simulink library "P45BPack_lib"  (R2025b)
settings: Solver=VariableStepAuto  StartTime=0.0  StopTime=10.0  RelTol=1e-3
values from neighbouring files (symbols this model uses):
  Np = evalin('base','Np')    [P45B.m]
  Ns = evalin('base','Ns')    [P45B.m]
undefined symbols (not defined in the file or in its folder): battery_builder_rtmsupport, gcbh, ModuleType1, ParallelAssemblyType1
libraries: nesl_utility x1, $bdroot x1
settings Model: Creator=nhamb  LastModifiedBy=nhamb

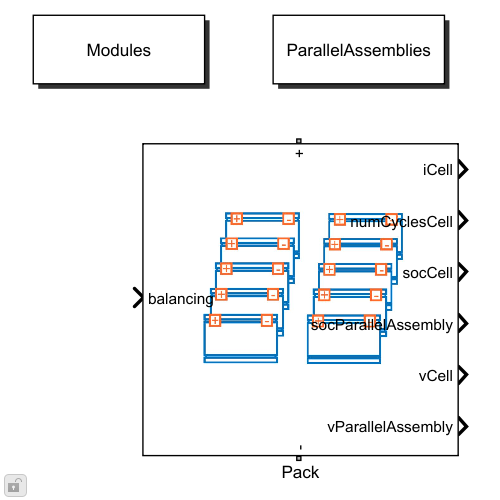
[thumbnail: Simulink's stored preview of the top-level diagram]
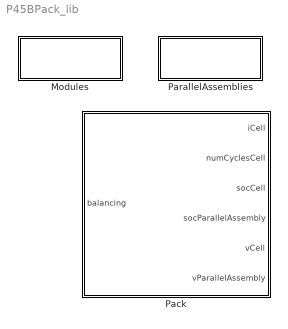
== system P45BPack_lib ==
  Modules : Subsystem  Tag=simscape_sublibrary
      mask Display: disp(get_param(gcb,'Name'))
  Pack : Subsystem  LoadFcn=battery_builder_rtmsupport('loadfcn',gcbh);
      settings: CopyFcn=battery_builder_rtmsupport('copyfcn',gcbh);  PreCopyFcn=battery_builder_rtmsupport('precopyfcn',gcbh);  PreDeleteFcn=battery_builder_rtmsupport('predeletefcn',gcbh);  PortSchema="{\"entries\":[{\"content\":{\"sides\":[{\"content\":{\"connectorIds\":[\"LConn1\"]},\"type\":\"ConnectorPlacement.EquallySpacedRectSide\",\"uuid\":\"bc69bedc-f021-4d63-9cf6-00df1ff9d80c\"},{\"content\":{\"connectorIds\":[\"RConn1\"],\"side\":\"RIGHT\"},\"type\":\"ConnectorPlacement.EquallySpacedRectSide\",\"uuid\":\"ae59a785-8ad2-4f04-8013-c306f8ca013b\"},{\"content\":{\"connectorIds\":[\"In1\"],\"side\":\"TOP\"},\"type\":\"ConnectorPlacement.EquallySpacedRectSide\",\"uuid\":\"2fb09327-c989-4719-8aff-5b8c99eb6fa6\"},{\"content\":{\"connectorIds\":[\"Out1\",\"Out2\",\"Out3\",\"Out4\",\"Out5\",\"Out6\"],\"side\":\"BOTTOM\"},\"type\":\"ConnectorPlacement.EquallySpacedRectSide\",\"uuid\":\"6b10cb86-7c8b-440d-835b-b9a65533e5ae\"}]},\"type\":\"ConnectorPlacement.EquallySpacedConnector\",\"uuid\":\"f3d89880-257d-496e-9c60-b9e40a370fad\"}],\"packageUris\":[\"http://schema.mathworks.com/mf0/Connector/R2020b\"],\"version\":\"1.0\"}"
      mask Display: image('$imagefile')
  ParallelAssemblies : Subsystem  Tag=simscape_sublibrary
      mask Display: disp(get_param(gcb,'Name'))

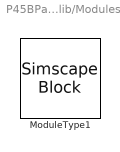
== system P45BPack_lib/Modules ==
  ModuleType1 : SimscapeBlock  DialogController=NetworkEngine.DynNeDlgSource  LoadFcn=|  SourceFile=P45BPack.Modules.ModuleType1  mask(ModuleType1){ComponentPath=P45BPack.Modules.ModuleType1, ComponentVariants=["P45BPack.Modules.ModuleType1"], ComponentVariantNames=["ModuleType1"], ClassName=ModuleType1, SchemaVersion=1, SOC_vecCell=ModuleType1.SOC_vecCell, SOC_vecCell_unit=1, SOC_vecCell_conf=compiletime, SOC_vecCellPercentDeviation=ModuleType1.SOC_vecCellPercentDeviation, SOC_vecCellPercentDeviation_unit=1, SOC_vecCellPercentDeviation_conf=compiletime, V0_vecCell=ModuleType1.V0_vecCell, V0_vecCell_unit=V, V0_vecCell_conf=compiletime, V0_vecCellPercentDeviation=ModuleType1.V0_vecCellPercentDeviation, V0_vecCellPercentDeviation_unit=1, V0_vecCellPercentDeviation_conf=compiletime, V_rangeCell=ModuleType1.V_rangeCell, V_rangeCell_unit=V, V_rangeCell_conf=compiletime, V_rangeCellPercentDeviation=ModuleType1.V_rangeCellPercentDeviation, V_rangeCellPercentDeviation_unit=1, V_rangeCellPercentDeviation_conf=compiletime, R0_vecCell=ModuleType1.R0_vecCell, R0_vecCell_unit=Ohm, R0_vecCell_conf=compiletime, R0_vecCellPercentDeviation=ModuleType1.R0_vecCellPercentDeviation, R0_vecCellPercentDeviation_unit=1, R0_vecCellPercentDeviation_conf=compiletime, AHCell=ModuleType1.AHCell, AHCell_unit=A*hr, AHCell_conf=compiletime, AHCellPercentDeviation=ModuleType1.AHCellPercentDeviation, AHCellPercentDeviation_unit=1, AHCellPercentDeviation_conf=compiletime, extrapolation_optionCell=simscape.enum.extrapolation.nearest, extrapolation_optionCell_unit=1, extrapolation_optionCell_conf=compiletime, R1_vecCell=ModuleType1.R1_vecCell, R1_vecCell_unit=Ohm, R1_vecCell_conf=compiletime, R1_vecCellPercentDeviation=ModuleType1.R1_vecCellPercentDeviation, R1_vecCellPercentDeviation_unit=1, R1_vecCellPercentDeviation_conf=compiletime, tau1_vecCell=ModuleType1.tau1_vecCell, tau1_vecCell_unit=s, tau1_vecCell_conf=compiletime, tau1_vecCellPercentDeviation=ModuleType1.tau1_vecCellPercentDeviation, tau1_vecCellPercentDeviation_unit=1, tau1_vecCellPercentDeviation_conf=compiletime, CellBalancingClosedResistance=ModuleType1.CellBalancingClosedResistance, CellBalancingClosedResistance_unit=Ohm, CellBalancingClosedResistance_conf=compiletime, CellBalancingOpenConductance=ModuleType1.CellBalancingOpenConductance, CellBalancingOpenConductance_unit=1/Ohm, CellBalancingOpenConductance_conf=compiletime, CellBalancingThreshold=ModuleType1.CellBalancingThreshold, CellBalancingThreshold_unit=1, CellBalancingThreshold_conf=compiletime, CellBalancingResistance=ModuleType1.CellBalancingResistance, CellBalancingResistance_unit=Ohm, CellBalancingResistance_conf=compiletime, P=2, P_unit=1, P_conf=compiletime, S=10, S_unit=1, S_conf=compiletime, iCell_specify=off, iCell_priority=None, iCell=repmat(0, 20, 1), iCell_unit=A, iCell_nominal_specify=off, iCell_nominal_value=1, iCell_nominal_unit=A, vCell_specify=off, vCell_priority=None, vCell=repmat(0, 20, 1), vCell_unit=V, vCell_nominal_specify=off, vCell_nominal_value=1, vCell_nominal_unit=V, socCell_specify=off, socCell_priority=High, socCell=repmat(1, 20, 1), socCell_unit=1, socCell_nominal_specify=off, socCell_nominal_value=1, socCell_nominal_unit=1, numCyclesCell_specify=off, numCyclesCell_priority=High, numCyclesCell=repmat(0, 20, 1), numCyclesCell_unit=1, numCyclesCell_nominal_specify=off, numCyclesCell_nominal_value=1, numCyclesCell_nominal_unit=1, vParallelAssembly_specify=off, vParallelAssembly_priority=None, vParallelAssembly=repmat(0, 10, 1), vParallelAssembly_unit=V, vParallelAssembly_nominal_specify=off, vParallelAssembly_nominal_value=1, vParallelAssembly_nominal_unit=V, socParallelAssembly_specify=off, socParallelAssembly_priority=None, socParallelAssembly=repmat(1, 10, 1), socParallelAssembly_unit=1, socParallelAssembly_nominal_specify=off, socParallelAssembly_nominal_value=1, socParallelAssembly_nominal_unit=1}
      | simscape.compiler.sli.internal.callback('LoadFcn',gcbh);
      | battery_builder_rtmsupport('loadfcn',gcbh);
      mask prompts: SOC_vecCell "Vector of state-of-charge values, SOC"; SOC_vecCellPercentDeviation "Percent deviation for SOC_vecCell"; V0_vecCell "Open-circuit voltage, V0(SOC)"; V0_vecCellPercentDeviation "Percent deviation for V0_vecCell"; V_rangeCell "Terminal voltage operating range [Min Max]"; V_rangeCellPercentDeviation "Percent deviation for V_rangeCell"; R0_vecCell "Terminal resistance, R0(SOC)"; R0_vecCellPercentDeviation "Percent deviation for R0_vecCell"; AHCell "Cell capacity, AH"; AHCellPercentDeviation "Percent deviation for AHCell"; extrapolation_optionCell "Extrapolation method for all tables"; R1_vecCell "First polarization resistance, R1(SOC)"; R1_vecCellPercentDeviation "Percent deviation for R1_vecCell"; tau1_vecCell "First time constant, tau1(SOC)"; tau1_vecCellPercentDeviation "Percent deviation for tau1_vecCell"; CellBalancingClosedResistance "Cell balancing switch closed resistance"; CellBalancingOpenConductance "Cell balancing switch open conductance"; CellBalancingThreshold "Cell balancing switch operation threshold"; CellBalancingResistance "Cell balancing shunt resistance"; P "Batteries in Parallel"; S "Batteries in Series"
      mask help:
      | Module Block
      |    Model resolution: Detailed
      |    Number of parallel assemblies: 10
      |    Number of cells per parallel assembly: 2
      |
      |    MATLAB version: 25.2
      |    Simscape Battery version: 25.2
      |    Simscape code generated on: 07-Sep-2026 17:43:40
      mask init:
      | simscape.compiler.sli.internal.preinitmask(gcb);
      settings: DeleteFcn=simscape.compiler.sli.internal.callback('DeleteFcn',gcbh);  ModelCloseFcn=simscape.compiler.sli.internal.callback('ModelCloseFcn',gcbh);  PreSaveFcn=simscape.compiler.sli.internal.callback('PreSaveFcn',gcbh);  PostSaveFcn=simscape.compiler.sli.internal.callback('PostSaveFcn',gcbh);  InternalSimscapePortConfiguration="{\"Bottom\":[{\"id\":\"n\",\"label\":\"-\",\"type\":\"foundation.electrical.electrical\"}],\"Left\":[{\"id\":\"enableCellBalancing\",\"label\":\"CB\",\"type\":\"input\"}],\"Right\":[],\"Top\":[{\"id\":\"p\",\"label\":\"+\",\"type\":\"foundation.electrical.electrical\"}]}"
      settings: CopyFcn=|
      | simscape.compiler.sli.internal.callback('CopyFcn',gcbh);
      | battery_builder_rtmsupport('copyfcn',gcbh);
      settings: PreCopyFcn=|
      | simscape.compiler.sli.internal.callback('PreCopyFcn',gcbh);
      | battery_builder_rtmsupport('precopyfcn',gcbh);
      settings: PreDeleteFcn=|
      | simscape.compiler.sli.internal.callback('PreDeleteFcn',gcbh);
      | battery_builder_rtmsupport('predeletefcn',gcbh);
      mask Help: web(nesl_help(gcbh))
      mask TypeOptions SOC_vecCell_unit: 1
      mask TypeOptions SOC_vecCell_conf: compiletime | runtime
      mask TypeOptions SOC_vecCellPercentDeviation_unit: 1
      mask TypeOptions SOC_vecCellPercentDeviation_conf: compiletime | runtime
      mask TypeOptions V0_vecCell_unit: V | MV | kV | mV
      mask TypeOptions V0_vecCell_conf: compiletime | runtime
      mask TypeOptions V0_vecCellPercentDeviation_unit: 1
      mask TypeOptions V0_vecCellPercentDeviation_conf: compiletime | runtime
      mask TypeOptions V_rangeCell_unit: V | MV | kV | mV
      mask TypeOptions V_rangeCell_conf: compiletime | runtime
      mask TypeOptions V_rangeCellPercentDeviation_unit: 1
      mask TypeOptions V_rangeCellPercentDeviation_conf: compiletime | runtime
      mask TypeOptions R0_vecCell_unit: Ohm | GOhm | MOhm | kOhm | mOhm
      mask TypeOptions R0_vecCell_conf: compiletime | runtime
      mask TypeOptions R0_vecCellPercentDeviation_unit: 1
      mask TypeOptions R0_vecCellPercentDeviation_conf: compiletime | runtime
      mask TypeOptions AHCell_unit: C | Ah | mC | nC | uC | MAh | kAh | mAh | A*hr
      mask TypeOptions AHCell_conf: compiletime | runtime
      mask TypeOptions AHCellPercentDeviation_unit: 1
      mask TypeOptions AHCellPercentDeviation_conf: compiletime | runtime
      mask TypeOptions extrapolation_optionCell: simscape.enum.extrapolation.linear | simscape.enum.extrapolation.nearest | simscape.enum.extrapolation.error
      mask TypeOptions extrapolation_optionCell_unit: 1
      mask TypeOptions extrapolation_optionCell_conf: compiletime
      mask TypeOptions R1_vecCell_unit: Ohm | GOhm | MOhm | kOhm | mOhm
      mask TypeOptions R1_vecCell_conf: compiletime | runtime
      mask TypeOptions R1_vecCellPercentDeviation_unit: 1
      mask TypeOptions R1_vecCellPercentDeviation_conf: compiletime | runtime
      mask TypeOptions tau1_vecCell_unit: d | s | hr | ms | ns | us | min
      mask TypeOptions tau1_vecCell_conf: compiletime | runtime
      mask TypeOptions tau1_vecCellPercentDeviation_unit: 1
      mask TypeOptions tau1_vecCellPercentDeviation_conf: compiletime | runtime
      mask TypeOptions CellBalancingClosedResistance_unit: Ohm | GOhm | MOhm | kOhm | mOhm
      mask TypeOptions CellBalancingClosedResistance_conf: compiletime | runtime
      mask TypeOptions CellBalancingOpenConductance_unit: S | mS | nS | uS | 1/Ohm
      mask TypeOptions CellBalancingOpenConductance_conf: compiletime | runtime
      mask TypeOptions CellBalancingThreshold_unit: 1
      mask TypeOptions CellBalancingThreshold_conf: compiletime | runtime
      mask TypeOptions CellBalancingResistance_unit: Ohm | GOhm | MOhm | kOhm | mOhm
      mask TypeOptions CellBalancingResistance_conf: compiletime | runtime
      mask TypeOptions P_unit: 1
      mask TypeOptions P_conf: compiletime
      mask TypeOptions S_unit: 1
      mask TypeOptions S_conf: compiletime
      mask TypeOptions iCell_priority: None | Low | High
      mask TypeOptions iCell_unit: A | MA | kA | mA | nA | pA | uA
      mask TypeOptions iCell_nominal_unit: A | MA | kA | mA | nA | pA | uA
      mask TypeOptions vCell_priority: None | Low | High
      mask TypeOptions vCell_unit: V | MV | kV | mV
      mask TypeOptions vCell_nominal_unit: V | MV | kV | mV
      mask TypeOptions socCell_priority: None | Low | High
      mask TypeOptions socCell_unit: 1
      mask TypeOptions socCell_nominal_unit: 1
      mask TypeOptions numCyclesCell_priority: None | Low | High
      mask TypeOptions numCyclesCell_unit: 1
      mask TypeOptions numCyclesCell_nominal_unit: 1
      mask TypeOptions vParallelAssembly_priority: None | Low | High
      mask TypeOptions vParallelAssembly_unit: V | MV | kV | mV
      mask TypeOptions vParallelAssembly_nominal_unit: V | MV | kV | mV
      mask TypeOptions socParallelAssembly_priority: None | Low | High
      mask TypeOptions socParallelAssembly_unit: 1
      mask TypeOptions socParallelAssembly_nominal_unit: 1
      mask DialogControl simscape__settings__group__ Prompt: physmod:common:gui:mli:schema:PISettingsTab
      mask DialogControl simscape__internal__group__name__1 Prompt: Main
      mask DialogControl simscape__internal__group__name__2 Prompt: Dynamics
      mask DialogControl simscape__internal__group__name__3 Prompt: Cell Balancing
      mask DialogControl simscape__internal__group__name__4 Prompt: Initial Targets
      mask DialogControl simscape__internal__group__name__5 Prompt: physmod:common:pi:sli:cs2ps:NominalContainer

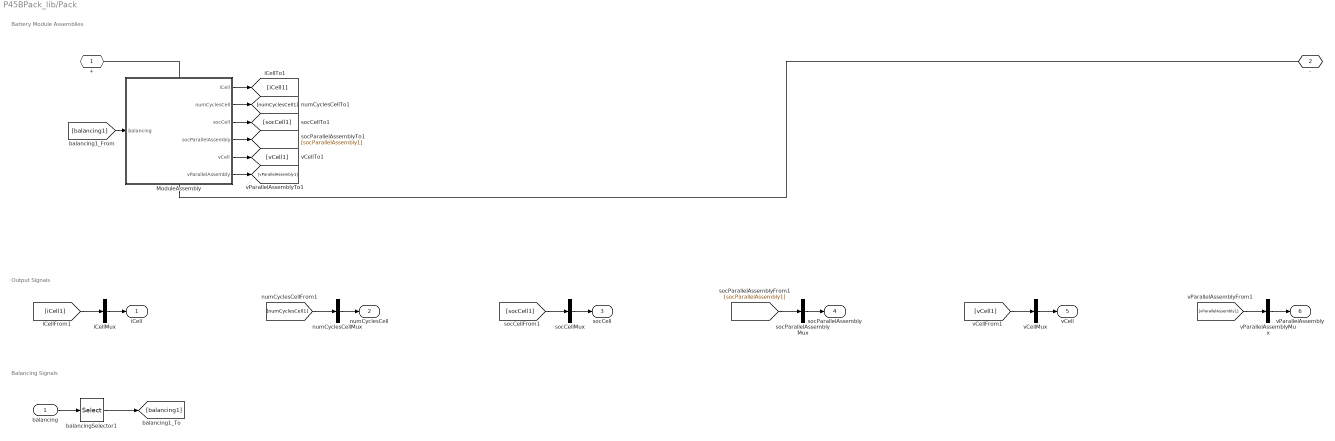
== system P45BPack_lib/Pack ==
  note: Balancing Signals
  note: Output Signals
  note: Battery Module Assemblies
  balancing : Inport  PortDimensions=Ns
  ModuleAssembly : Subsystem  LoadFcn=battery_builder_rtmsupport('loadfcn',gcbh);
      settings: CopyFcn=battery_builder_rtmsupport('copyfcn',gcbh);  PreCopyFcn=battery_builder_rtmsupport('precopyfcn',gcbh);  PreDeleteFcn=battery_builder_rtmsupport('predeletefcn',gcbh);  PortSchema="{\"entries\":[{\"content\":{\"sides\":[{\"content\":{\"connectorIds\":[\"LConn1\"]},\"type\":\"ConnectorPlacement.EquallySpacedRectSide\",\"uuid\":\"bc69bedc-f021-4d63-9cf6-00df1ff9d80c\"},{\"content\":{\"connectorIds\":[\"RConn1\"],\"side\":\"RIGHT\"},\"type\":\"ConnectorPlacement.EquallySpacedRectSide\",\"uuid\":\"ae59a785-8ad2-4f04-8013-c306f8ca013b\"},{\"content\":{\"connectorIds\":[\"In1\"],\"side\":\"TOP\"},\"type\":\"ConnectorPlacement.EquallySpacedRectSide\",\"uuid\":\"2fb09327-c989-4719-8aff-5b8c99eb6fa6\"},{\"content\":{\"connectorIds\":[\"Out1\",\"Out2\",\"Out3\",\"Out4\",\"Out5\",\"Out6\"],\"side\":\"BOTTOM\"},\"type\":\"ConnectorPlacement.EquallySpacedRectSide\",\"uuid\":\"26742bc9-9886-4824-abba-948048412869\"}]},\"type\":\"ConnectorPlacement.EquallySpacedConnector\",\"uuid\":\"f3d89880-257d-496e-9c60-b9e40a370fad\"}],\"packageUris\":[\"http://schema.mathworks.com/mf0/Connector/R2020b\"],\"version\":\"1.0\"}"
      mask Display: image('$imagefile')
  balancingSelector1 : Selector  InputPortWidth=Ns  IndexOptions=Index vector (dialog)  Indices=1:Ns  OutputSizes=1
  iCellMux : Mux  Inputs=1
  numCyclesCellMux : Mux  Inputs=1
  socCellMux : Mux  Inputs=1
  socParallelAssemblyMux : Mux  Inputs=1
  vCellMux : Mux  Inputs=1
  vParallelAssemblyMux : Mux  Inputs=1
  + : PMIOPort  Side=Left
  - : PMIOPort  Port=2  Side=Right
  iCell : Outport
  numCyclesCell : Outport  Port=2
  socCell : Outport  Port=3
  socParallelAssembly : Outport  Port=4
  vCell : Outport  Port=5
  vParallelAssembly : Outport  Port=6
  wires:
  balancingSelector1/1 -> [balancing1]
  balancing/1 -> balancingSelector1/1
  [balancing1] -> ModuleAssembly/1(balancing)
  [vParallelAssembly1] -> vParallelAssemblyMux/1
  vParallelAssemblyMux/1 -> vParallelAssembly/1
  ModuleAssembly/6(vParallelAssembly) -> [vParallelAssembly1]
  [vCell1] -> vCellMux/1
  vCellMux/1 -> vCell/1
  ModuleAssembly/5(vCell) -> [vCell1]
  [socParallelAssembly1] -> socParallelAssemblyMux/1
  socParallelAssemblyMux/1 -> socParallelAssembly/1
  ModuleAssembly/4(socParallelAssembly) -> [socParallelAssembly1]
  [socCell1] -> socCellMux/1
  socCellMux/1 -> socCell/1
  ModuleAssembly/3(socCell) -> [socCell1]
  [numCyclesCell1] -> numCyclesCellMux/1
  numCyclesCellMux/1 -> numCyclesCell/1
  ModuleAssembly/2(numCyclesCell) -> [numCyclesCell1]
  [iCell1] -> iCellMux/1
  iCellMux/1 -> iCell/1
  ModuleAssembly/1(iCell) -> [iCell1]
  connections:
  ModuleAssembly/RConn1 -- -/RConn1
  ModuleAssembly/LConn1 -- +/RConn1

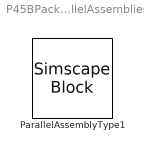
== system P45BPack_lib/ParallelAssemblies ==
  ParallelAssemblyType1 : SimscapeBlock  DialogController=NetworkEngine.DynNeDlgSource  LoadFcn=|  SourceFile=P45BPack.ParallelAssemblies.ParallelAssemblyType1  mask(ParallelAssemblyType1){ComponentPath=P45BPack.ParallelAssemblies.ParallelAssemblyType1, ComponentVariants=["P45BPack.ParallelAssemblies.ParallelAssemblyType1"], ComponentVariantNames=["ParallelAssemblyType1"], ClassName=ParallelAssemblyType1, SchemaVersion=1, SOC_vecCell=ParallelAssemblyType1.SOC_vecCell, SOC_vecCell_unit=1, SOC_vecCell_conf=compiletime, SOC_vecCellPercentDeviation=ParallelAssemblyType1.SOC_vecCellPercentDeviation, SOC_vecCellPercentDeviation_unit=1, SOC_vecCellPercentDeviation_conf=compiletime, V0_vecCell=ParallelAssemblyType1.V0_vecCell, V0_vecCell_unit=V, V0_vecCell_conf=compiletime, V0_vecCellPercentDeviation=ParallelAssemblyType1.V0_vecCellPercentDeviation, V0_vecCellPercentDeviation_unit=1, V0_vecCellPercentDeviation_conf=compiletime, V_rangeCell=ParallelAssemblyType1.V_rangeCell, V_rangeCell_unit=V, V_rangeCell_conf=compiletime, V_rangeCellPercentDeviation=ParallelAssemblyType1.V_rangeCellPercentDeviation, V_rangeCellPercentDeviation_unit=1, V_rangeCellPercentDeviation_conf=compiletime, R0_vecCell=ParallelAssemblyType1.R0_vecCell, R0_vecCell_unit=Ohm, R0_vecCell_conf=compiletime, R0_vecCellPercentDeviation=ParallelAssemblyType1.R0_vecCellPercentDeviation, R0_vecCellPercentDeviation_unit=1, R0_vecCellPercentDeviation_conf=compiletime, AHCell=ParallelAssemblyType1.AHCell, AHCell_unit=A*hr, AHCell_conf=compiletime, AHCellPercentDeviation=ParallelAssemblyType1.AHCellPercentDeviation, AHCellPercentDeviation_unit=1, AHCellPercentDeviation_conf=compiletime, extrapolation_optionCell=simscape.enum.extrapolation.nearest, extrapolation_optionCell_unit=1, extrapolation_optionCell_conf=compiletime, R1_vecCell=ParallelAssemblyType1.R1_vecCell, R1_vecCell_unit=Ohm, R1_vecCell_conf=compiletime, R1_vecCellPercentDeviation=ParallelAssemblyType1.R1_vecCellPercentDeviation, R1_vecCellPercentDeviation_unit=1, R1_vecCellPercentDeviation_conf=compiletime, tau1_vecCell=ParallelAssemblyType1.tau1_vecCell, tau1_vecCell_unit=s, tau1_vecCell_conf=compiletime, tau1_vecCellPercentDeviation=ParallelAssemblyType1.tau1_vecCellPercentDeviation, tau1_vecCellPercentDeviation_unit=1, tau1_vecCellPercentDeviation_conf=compiletime, CellBalancingClosedResistance=ParallelAssemblyType1.CellBalancingClosedResistance, CellBalancingClosedResistance_unit=Ohm, CellBalancingClosedResistance_conf=compiletime, CellBalancingOpenConductance=ParallelAssemblyType1.CellBalancingOpenConductance, CellBalancingOpenConductance_unit=1/Ohm, CellBalancingOpenConductance_conf=compiletime, CellBalancingThreshold=ParallelAssemblyType1.CellBalancingThreshold, CellBalancingThreshold_unit=1, CellBalancingThreshold_conf=compiletime, CellBalancingResistance=ParallelAssemblyType1.CellBalancingResistance, CellBalancingResistance_unit=Ohm, CellBalancingResistance_conf=compiletime, P=2, P_unit=1, P_conf=compiletime, iCell_specify=off, iCell_priority=None, iCell=repmat(0, 2, 1), iCell_unit=A, iCell_nominal_specify=off, iCell_nominal_value=1, iCell_nominal_unit=A, vCell_specify=off, vCell_priority=None, vCell=repmat(0, 2, 1), vCell_unit=V, vCell_nominal_specify=off, vCell_nominal_value=1, vCell_nominal_unit=V, socCell_specify=off, socCell_priority=High, socCell=repmat(1, 2, 1), socCell_unit=1, socCell_nominal_specify=off, socCell_nominal_value=1, socCell_nominal_unit=1, numCyclesCell_specify=off, numCyclesCell_priority=High, numCyclesCell=repmat(0, 2, 1), numCyclesCell_unit=1, numCyclesCell_nominal_specify=off, numCyclesCell_nominal_value=1, numCyclesCell_nominal_unit=1, vParallelAssembly_specify=off, vParallelAssembly_priority=None, vParallelAssembly=0, vParallelAssembly_unit=V, vParallelAssembly_nominal_specify=off, vParallelAssembly_nominal_value=1, vParallelAssembly_nominal_unit=V, socParallelAssembly_specify=off, socParallelAssembly_priority=None, socParallelAssembly=1, socParallelAssembly_unit=1, socParallelAssembly_nominal_specify=off, socParallelAssembly_nominal_value=1, socParallelAssembly_nominal_unit=1}
      | simscape.compiler.sli.internal.callback('LoadFcn',gcbh);
      | battery_builder_rtmsupport('loadfcn',gcbh);
      mask prompts: SOC_vecCell "Vector of state-of-charge values, SOC"; SOC_vecCellPercentDeviation "Percent deviation for SOC_vecCell"; V0_vecCell "Open-circuit voltage, V0(SOC)"; V0_vecCellPercentDeviation "Percent deviation for V0_vecCell"; V_rangeCell "Terminal voltage operating range [Min Max]"; V_rangeCellPercentDeviation "Percent deviation for V_rangeCell"; R0_vecCell "Terminal resistance, R0(SOC)"; R0_vecCellPercentDeviation "Percent deviation for R0_vecCell"; AHCell "Cell capacity, AH"; AHCellPercentDeviation "Percent deviation for AHCell"; extrapolation_optionCell "Extrapolation method for all tables"; R1_vecCell "First polarization resistance, R1(SOC)"; R1_vecCellPercentDeviation "Percent deviation for R1_vecCell"; tau1_vecCell "First time constant, tau1(SOC)"; tau1_vecCellPercentDeviation "Percent deviation for tau1_vecCell"; CellBalancingClosedResistance "Cell balancing switch closed resistance"; CellBalancingOpenConductance "Cell balancing switch open conductance"; CellBalancingThreshold "Cell balancing switch operation threshold"; CellBalancingResistance "Cell balancing shunt resistance"; P "Batteries in Parallel"
      mask help:
      | Parallel Assembly Block
      |    Model resolution: Detailed
      |    Number of cells: 2
      |
      |    MATLAB version: 25.2
      |    Simscape Battery version: 25.2
      |    Simscape code generated on: 07-Sep-2026 17:43:39
      mask init:
      | simscape.compiler.sli.internal.preinitmask(gcb);
      settings: DeleteFcn=simscape.compiler.sli.internal.callback('DeleteFcn',gcbh);  ModelCloseFcn=simscape.compiler.sli.internal.callback('ModelCloseFcn',gcbh);  PreSaveFcn=simscape.compiler.sli.internal.callback('PreSaveFcn',gcbh);  PostSaveFcn=simscape.compiler.sli.internal.callback('PostSaveFcn',gcbh);  InternalSimscapePortConfiguration="{\"Bottom\":[{\"id\":\"n\",\"label\":\"-\",\"type\":\"foundation.electrical.electrical\"}],\"Left\":[{\"id\":\"enableCellBalancing\",\"label\":\"CB\",\"type\":\"input\"}],\"Right\":[],\"Top\":[{\"id\":\"p\",\"label\":\"+\",\"type\":\"foundation.electrical.electrical\"}]}"
      settings: CopyFcn=|
      | simscape.compiler.sli.internal.callback('CopyFcn',gcbh);
      | battery_builder_rtmsupport('copyfcn',gcbh);
      settings: PreCopyFcn=|
      | simscape.compiler.sli.internal.callback('PreCopyFcn',gcbh);
      | battery_builder_rtmsupport('precopyfcn',gcbh);
      settings: PreDeleteFcn=|
      | simscape.compiler.sli.internal.callback('PreDeleteFcn',gcbh);
      | battery_builder_rtmsupport('predeletefcn',gcbh);
      mask Help: web(nesl_help(gcbh))
      mask TypeOptions SOC_vecCell_unit: 1
      mask TypeOptions SOC_vecCell_conf: compiletime | runtime
      mask TypeOptions SOC_vecCellPercentDeviation_unit: 1
      mask TypeOptions SOC_vecCellPercentDeviation_conf: compiletime | runtime
      mask TypeOptions V0_vecCell_unit: V | MV | kV | mV
      mask TypeOptions V0_vecCell_conf: compiletime | runtime
      mask TypeOptions V0_vecCellPercentDeviation_unit: 1
      mask TypeOptions V0_vecCellPercentDeviation_conf: compiletime | runtime
      mask TypeOptions V_rangeCell_unit: V | MV | kV | mV
      mask TypeOptions V_rangeCell_conf: compiletime | runtime
      mask TypeOptions V_rangeCellPercentDeviation_unit: 1
      mask TypeOptions V_rangeCellPercentDeviation_conf: compiletime | runtime
      mask TypeOptions R0_vecCell_unit: Ohm | GOhm | MOhm | kOhm | mOhm
      mask TypeOptions R0_vecCell_conf: compiletime | runtime
      mask TypeOptions R0_vecCellPercentDeviation_unit: 1
      mask TypeOptions R0_vecCellPercentDeviation_conf: compiletime | runtime
      mask TypeOptions AHCell_unit: C | Ah | mC | nC | uC | MAh | kAh | mAh | A*hr
      mask TypeOptions AHCell_conf: compiletime | runtime
      mask TypeOptions AHCellPercentDeviation_unit: 1
      mask TypeOptions AHCellPercentDeviation_conf: compiletime | runtime
      mask TypeOptions extrapolation_optionCell: simscape.enum.extrapolation.linear | simscape.enum.extrapolation.nearest | simscape.enum.extrapolation.error
      mask TypeOptions extrapolation_optionCell_unit: 1
      mask TypeOptions extrapolation_optionCell_conf: compiletime
      mask TypeOptions R1_vecCell_unit: Ohm | GOhm | MOhm | kOhm | mOhm
      mask TypeOptions R1_vecCell_conf: compiletime | runtime
      mask TypeOptions R1_vecCellPercentDeviation_unit: 1
      mask TypeOptions R1_vecCellPercentDeviation_conf: compiletime | runtime
      mask TypeOptions tau1_vecCell_unit: d | s | hr | ms | ns | us | min
      mask TypeOptions tau1_vecCell_conf: compiletime | runtime
      mask TypeOptions tau1_vecCellPercentDeviation_unit: 1
      mask TypeOptions tau1_vecCellPercentDeviation_conf: compiletime | runtime
      mask TypeOptions CellBalancingClosedResistance_unit: Ohm | GOhm | MOhm | kOhm | mOhm
      mask TypeOptions CellBalancingClosedResistance_conf: compiletime | runtime
      mask TypeOptions CellBalancingOpenConductance_unit: S | mS | nS | uS | 1/Ohm
      mask TypeOptions CellBalancingOpenConductance_conf: compiletime | runtime
      mask TypeOptions CellBalancingThreshold_unit: 1
      mask TypeOptions CellBalancingThreshold_conf: compiletime | runtime
      mask TypeOptions CellBalancingResistance_unit: Ohm | GOhm | MOhm | kOhm | mOhm
      mask TypeOptions CellBalancingResistance_conf: compiletime | runtime
      mask TypeOptions P_unit: 1
      mask TypeOptions P_conf: compiletime
      mask TypeOptions iCell_priority: None | Low | High
      mask TypeOptions iCell_unit: A | MA | kA | mA | nA | pA | uA
      mask TypeOptions iCell_nominal_unit: A | MA | kA | mA | nA | pA | uA
      mask TypeOptions vCell_priority: None | Low | High
      mask TypeOptions vCell_unit: V | MV | kV | mV
      mask TypeOptions vCell_nominal_unit: V | MV | kV | mV
      mask TypeOptions socCell_priority: None | Low | High
      mask TypeOptions socCell_unit: 1
      mask TypeOptions socCell_nominal_unit: 1
      mask TypeOptions numCyclesCell_priority: None | Low | High
      mask TypeOptions numCyclesCell_unit: 1
      mask TypeOptions numCyclesCell_nominal_unit: 1
      mask TypeOptions vParallelAssembly_priority: None | Low | High
      mask TypeOptions vParallelAssembly_unit: V | MV | kV | mV
      mask TypeOptions vParallelAssembly_nominal_unit: V | MV | kV | mV
      mask TypeOptions socParallelAssembly_priority: None | Low | High
      mask TypeOptions socParallelAssembly_unit: 1
      mask TypeOptions socParallelAssembly_nominal_unit: 1
      mask DialogControl simscape__settings__group__ Prompt: physmod:common:gui:mli:schema:PISettingsTab
      mask DialogControl simscape__internal__group__name__1 Prompt: Main
      mask DialogControl simscape__internal__group__name__2 Prompt: Dynamics
      mask DialogControl simscape__internal__group__name__3 Prompt: Cell Balancing
      mask DialogControl simscape__internal__group__name__4 Prompt: Initial Targets
      mask DialogControl simscape__internal__group__name__5 Prompt: physmod:common:pi:sli:cs2ps:NominalContainer

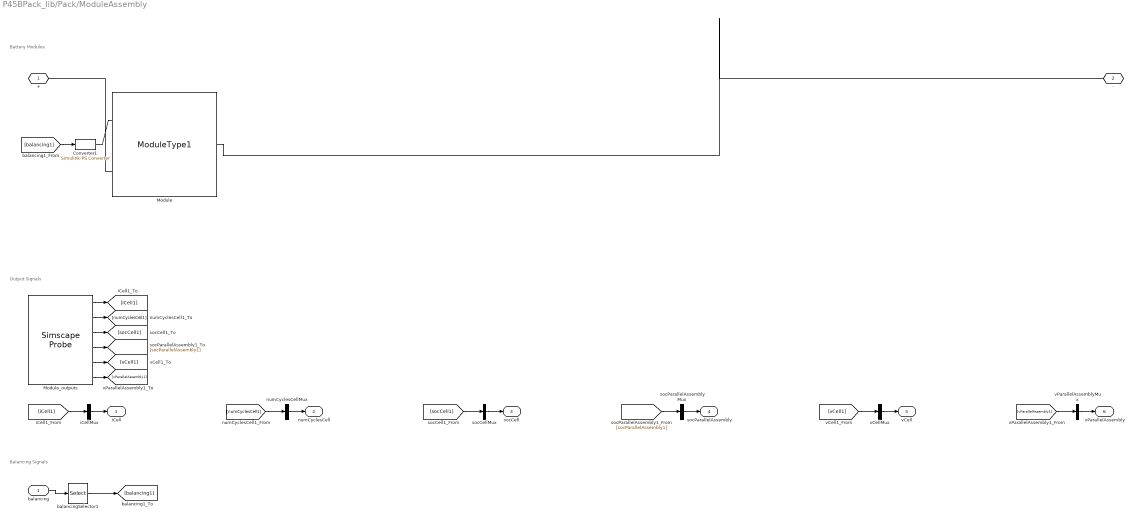
== system P45BPack_lib/Pack/ModuleAssembly ==
  note: Battery Modules
  note: Output Signals
  note: Balancing Signals
  balancing : Inport  PortDimensions=Ns
  Converter1 : nesl_utility/Simulink-PS Converter  PhysicalDomain=network_engine_domain  SubClassName=ps_input  LeftPortType=input  RightPortType=output  PseudoPeriodic=off  Frequencies=[]  NoiseDistribution=none  NoiseParameters=[]  Unit=1  AffineConversion=off  FilteringAndDerivatives=provide  SimscapeFilterOrder=1  InputFilterTimeConstant=0.001  UdotUserProvided=0
  Module : $bdroot/Modules/ModuleType1  SOC_vecCell=Pack.SOC_vecCell  SOC_vecCellPercentDeviation=Pack.SOC_vecCellPercentDeviation  V0_vecCell=Pack.V0_vecCell V  V0_vecCellPercentDeviation=Pack.V0_vecCellPercentDeviation  V_rangeCell=Pack.V_rangeCell V  V_rangeCellPercentDeviation=Pack.V_rangeCellPercentDeviation  R0_vecCell=Pack.R0_vecCell Ohm  R0_vecCellPercentDeviation=Pack.R0_vecCellPercentDeviation  AHCell=Pack.AHCell A*hr  AHCellPercentDeviation=Pack.AHCellPercentDeviation  extrapolation_optionCell=simscape.enum.extrapolation.nearest  R1_vecCell=Pack.R1_vecCell Ohm  R1_vecCellPercentDeviation=Pack.R1_vecCellPercentDeviation  tau1_vecCell=Pack.tau1_vecCell s  tau1_vecCellPercentDeviation=Pack.tau1_vecCellPercentDeviation  CellBalancingClosedResistance=Pack.CellBalancingClosedResistance Ohm  CellBalancingOpenConductance=Pack.CellBalancingOpenConductance 1/Ohm  CellBalancingThreshold=Pack.CellBalancingThreshold  CellBalancingResistance=Pack.CellBalancingResistance Ohm  P=Np  S=Ns  iCell_specify=off  iCell_priority=None  iCell=repmat(0, 20, 1) A  iCell_nominal_specify=off  iCell_nominal_value=1  iCell_nominal_unit=A  vCell_specify=off  vCell_priority=None  vCell=repmat(0, 20, 1) V  vCell_nominal_specify=off  vCell_nominal_value=1  vCell_nominal_unit=V  socCell_specify=on  socCell_priority=High  socCell=SOC0Cell  socCell_nominal_specify=off  socCell_nominal_value=1  socCell_nominal_unit=1  numCyclesCell_specify=off  numCyclesCell_priority=High  numCyclesCell=repmat(0, 20, 1)  numCyclesCell_nominal_specify=off  numCyclesCell_nominal_value=1  numCyclesCell_nominal_unit=1  vParallelAssembly_specify=off  vParallelAssembly_priority=None  vParallelAssembly=repmat(0, 10, 1) V  vParallelAssembly_nominal_specify=off  vParallelAssembly_nominal_value=1  vParallelAssembly_nominal_unit=V  socParallelAssembly_specify=off  socParallelAssembly_priority=None  socParallelAssembly=repmat(1, 10, 1)  socParallelAssembly_nominal_specify=off  socParallelAssembly_nominal_value=1  socParallelAssembly_nominal_unit=1
      settings: InternalSimscapePortConfiguration="{\"Bottom\":[{\"id\":\"n\",\"label\":\"-\",\"type\":\"foundation.electrical.electrical\"}],\"Left\":[{\"id\":\"enableCellBalancing\",\"label\":\"CB\",\"type\":\"input\"}],\"Right\":[],\"Top\":[{\"id\":\"p\",\"label\":\"+\",\"type\":\"foundation.electrical.electrical\"}]}"
  Module_outputs : SimscapeProbe  BoundBlock=10  Variables="{\"iCell\":{\"Probing\":\"ON\"},\"numCyclesCell\":{\"Probing\":\"ON\"},\"socCell\":{\"Probing\":\"ON\"},\"socParallelAssembly\":{\"Probing\":\"ON\"},\"vCell\":{\"Probing\":\"ON\"},\"vParallelAssembly\":{\"Probing\":\"ON\"}}"
  balancingSelector1 : Selector  InputPortWidth=Ns  IndexOptions=Index vector (dialog)  Indices=1:Ns  OutputSizes=1
  iCellMux : Mux  Inputs=1
  numCyclesCellMux : Mux  Inputs=1
  socCellMux : Mux  Inputs=1
  socParallelAssemblyMux : Mux  Inputs=1
  vCellMux : Mux  Inputs=1
  vParallelAssemblyMux : Mux  Inputs=1
  + : PMIOPort  Side=Left
  - : PMIOPort  Port=2  Side=Right
  iCell : Outport
  numCyclesCell : Outport  Port=2
  socCell : Outport  Port=3
  socParallelAssembly : Outport  Port=4
  vCell : Outport  Port=5
  vParallelAssembly : Outport  Port=6
  wires:
  Module_outputs/1 -> [iCell1]
  iCellMux/1 -> iCell/1
  [iCell1] -> iCellMux/1
  Module_outputs/2 -> [numCyclesCell1]
  numCyclesCellMux/1 -> numCyclesCell/1
  [numCyclesCell1] -> numCyclesCellMux/1
  Module_outputs/3 -> [socCell1]
  socCellMux/1 -> socCell/1
  [socCell1] -> socCellMux/1
  Module_outputs/4 -> [socParallelAssembly1]
  socParallelAssemblyMux/1 -> socParallelAssembly/1
  [socParallelAssembly1] -> socParallelAssemblyMux/1
  Module_outputs/5 -> [vCell1]
  vCellMux/1 -> vCell/1
  [vCell1] -> vCellMux/1
  Module_outputs/6 -> [vParallelAssembly1]
  vParallelAssemblyMux/1 -> vParallelAssembly/1
  [vParallelAssembly1] -> vParallelAssemblyMux/1
  [balancing1] -> Converter1/1
  balancing/1 -> balancingSelector1/1
  balancingSelector1/1 -> [balancing1]
  connections:
  Module/LConn2 -- +/RConn1
  Module/RConn1 -- -/RConn1
  Converter1/RConn1 -- Module/LConn1
